simulink model "ride_model"  (R2019a)
settings: Solver=VariableStepAuto  StartTime=0.0  StopTime=120  RelTol=1e-3
libraries: fl_lib x20, nesl_utility x10, eeGeneralControl x1, sdl_lib x1
settings Model: Creator=Owen Heaney  LastModifiedBy=Owen Heaney

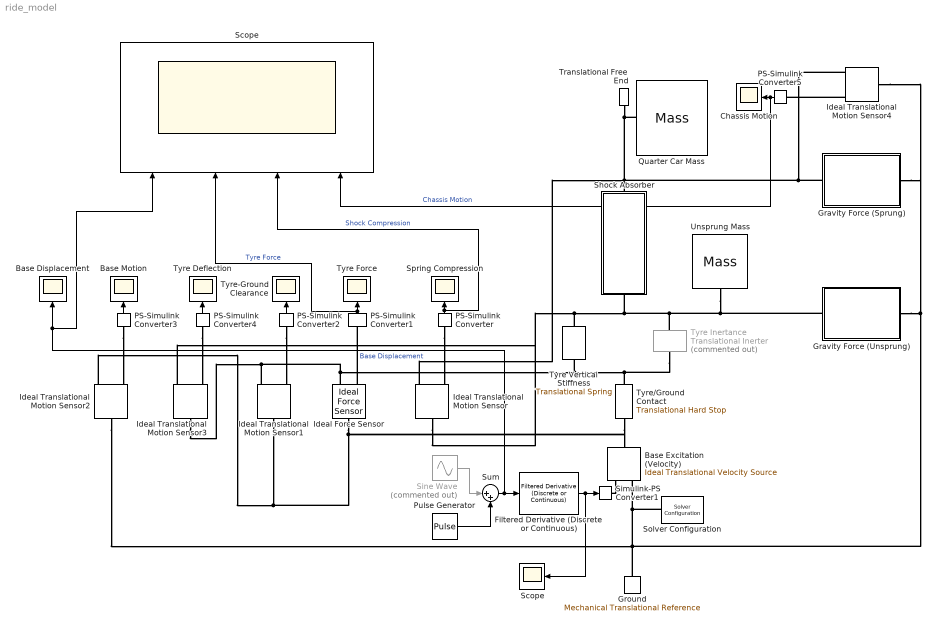
== system ride_model ==
  " Scope" : Scope  NumInputPorts=4
  Base Displacement : Scope
  Base Motion : Scope
  Base Excitation (Velocity) : fl_lib/Mechanical/Mechanical Sources/Ideal Translational Velocity Source
  Chassis Motion : Scope
  Filtered Derivative (Discrete or Continuous) : eeGeneralControl/Filtered Derivative (Discrete or Continuous)  K=1  T=0.0001  B=inf  A=-inf  minRatio=10  Ts=0
      settings: SourceProductName=Simscape Electrical  SourceProductBaseCode=PS
  Gravity Force (Sprung) : Subsystem
  Gravity Force (Unsprung) : Subsystem
  Ground : fl_lib/Mechanical/Translational Elements/Mechanical Translational Reference
  Ideal Force Sensor : fl_lib/Mechanical/Mechanical Sensors/Ideal Force Sensor
  Ideal Translational Motion Sensor{,1..4} (5 alike) : fl_lib/Mechanical/Mechanical Sensors/Ideal Translational Motion Sensor  offset=0 m
  PS-Simulink Converter : nesl_utility/PS-Simulink Converter  PhysicalDomain=network_engine_domain  SubClassName=ps_output  LeftPortType=input  RightPortType=output  PseudoPeriodic=off  Frequencies=[]  Unit=mm  AffineConversion=off
  PS-Simulink Converter{1..4} (4 alike) : nesl_utility/PS-Simulink Converter  PhysicalDomain=network_engine_domain  SubClassName=ps_output  LeftPortType=input  RightPortType=output  PseudoPeriodic=off  Frequencies=[]  Unit=1  AffineConversion=off
  PS-Simulink Converter5 : nesl_utility/PS-Simulink Converter  PhysicalDomain=network_engine_domain  SubClassName=ps_output  LeftPortType=input  RightPortType=output  PseudoPeriodic=off  Frequencies=[]  Unit=mm  AffineConversion=off
  Pulse Generator : DiscretePulseGenerator  PulseType=Time based  Amplitude=0.002  Period=60  PulseWidth=25  PhaseDelay=20
  Quarter Car Mass : fl_lib/Mechanical/Translational Elements/Mass  mass=75 kg  v_specify=off  v_priority=High  v=0 m/s  v_nominal_specify=off  v_nominal_unit=m/s  v_nominal_value=1  f_specify=on  f_priority=None  f=0.01 N  f_nominal_specify=off  f_nominal_unit=N  f_nominal_value=1
  Scope : Scope
  Shock Absorber : Subsystem
  Simulink-PS Converter1 : nesl_utility/Simulink-PS Converter  PhysicalDomain=network_engine_domain  SubClassName=ps_input  LeftPortType=input  RightPortType=output  PseudoPeriodic=off  Frequencies=[]  NoiseDistribution=none  NoiseParameters=[]  Unit=m/s  AffineConversion=off  FilteringAndDerivatives=filter  SimscapeFilterOrder=1  InputFilterTimeConstant=0.001  UdotUserProvided=0
  Sine Wave : Sin  Commented=on  Amplitude=0.001  Frequency=5  SampleTime=0
  Solver Configuration : nesl_utility/Solver Configuration  PhysicalDomain=network_engine_domain  SubClassName=solver  LeftPortType=input  RightPortType=generic  Tones=[]  Harmonics=[]  SimulateNoise=off  Profile=off  UseLocalSampling=off  EnableSwitchedLinearOptims=on  FrequencyDomain=off  UseCCode=off  RelTol=0.001  AbsTol=1e-06  MinStep=1e-09  ToWorkspace=off  RevertToSquareIcSolve=off  NumHomotopyIterations=100  PhasorMode=off  PhasorModeNumHarmonics=1  DoDC=on  ResidualTolerance=1e-15  UseLocalSolver=off  LocalSolverChoice=NE_BACKWARD_EULER_ADVANCER  LocalSolverSampleTime=0.001  DoFixedCost=off  MaxNonlinIter=3  MaxModeIter=2  LinearAlgebra=auto  EquationFormulation=NE_TIME_EF  DelaysMemoryBudget=1024  AutomaticFiltering=on  FilteringTimeConstant=0.001  PartitionStorageMethod=AS_NEEDED  PartitionMemoryBudget=1024  PartitionMethod=ROBUST
  Spring Compression : Scope
  Sum : Sum  Inputs=|++
  Translational Free End : fl_lib/Mechanical/Translational Elements/Translational Free End  v_specify=off  v_priority=None  v=0 m/s  v_nominal_specify=off  v_nominal_unit=m/s  v_nominal_value=1
      settings: SourceProductName=Simscape  SourceProductBaseCode=SS
  Tyre Deflection : Scope
  Tyre Force : Scope
  Tyre Inertance : fl_lib/Mechanical/Translational Elements/Translational Inerter  Commented=on  B=0.001 kg  v_specify=off  v_priority=High  v=0 m/s  v_nominal_specify=off  v_nominal_unit=m/s  v_nominal_value=1  f_specify=off  f_priority=None  f=0 N  f_nominal_specify=off  f_nominal_unit=N  f_nominal_value=1
      settings: SourceProductName=Simscape  SourceProductBaseCode=SS
  Tyre Vertical Stiffness : fl_lib/Mechanical/Translational Elements/Translational Spring  spr_rate=80000 N/m  v_specify=on  v_priority=None  v=0 m/s  v_nominal_specify=off  v_nominal_unit=m/s  v_nominal_value=1  f_specify=off  f_priority=None  f=0 N  f_nominal_specify=off  f_nominal_unit=N  f_nominal_value=1  x_specify=off  x_priority=High  x=0 m  x_nominal_specify=off  x_nominal_unit=m  x_nominal_value=1
  Tyre-Ground Clearance : Scope
  Tyre/Ground Contact : fl_lib/Mechanical/Translational Elements/Translational Hard Stop  upper_bnd=100 m  lower_bnd=0 mm  stiff_up=inf N/m  stiff_low=inf N/m  D_up=inf N/(m/s)  D_low=0 N/(m/s)  model=simscape.enum.hardstop.fullundamped  transition=00.1 mm  v_specify=off  v_priority=None  v=0 m/s  v_nominal_specify=off  v_nominal_unit=m/s  v_nominal_value=1  f_specify=off  f_priority=None  f=0 N  f_nominal_specify=off  f_nominal_unit=N  f_nominal_value=1  x_specify=off  x_priority=High  x=0 m  x_nominal_specify=off  x_nominal_unit=m  x_nominal_value=1
  Unsprung Mass : fl_lib/Mechanical/Translational Elements/Mass  mass=5 kg  v_specify=off  v_priority=High  v=0 m/s  v_nominal_specify=off  v_nominal_unit=m/s  v_nominal_value=1  f_specify=on  f_priority=None  f=-0.01 N  f_nominal_specify=off  f_nominal_unit=N  f_nominal_value=1
  wires:
  PS-Simulink Converter/1 -> " Scope"/3, Spring Compression/1  "Shock Compression"
  PS-Simulink Converter1/1 -> " Scope"/2, Tyre Force/1  "Tyre Force"
  PS-Simulink Converter2/1 -> Tyre-Ground Clearance/1
  PS-Simulink Converter3/1 -> Base Motion/1
  PS-Simulink Converter4/1 -> Tyre Deflection/1
  Filtered Derivative (Discrete or Continuous)/1 -> Scope/1, Simulink-PS Converter1/1
  Sum/1 -> " Scope"/1, Base Displacement/1, Filtered Derivative (Discrete or Continuous)/1  "Base Displacement"
  Pulse Generator/1 -> Sum/2
  Sine Wave/1 -> Sum/1
  PS-Simulink Converter5/1 -> " Scope"/4, Chassis Motion/1  "Chassis Motion"
  connections:
  Gravity Force (Sprung)/LConn1 -- Ideal Translational Motion Sensor4/RConn1 -- Shock Absorber/LConn1 -- Ideal Translational Motion Sensor/RConn1 -- Translational Free End/LConn1 -- Quarter Car Mass/LConn1
  Ideal Translational Motion Sensor2/LConn1 -- Ground/LConn1 -- Ideal Translational Motion Sensor4/LConn1 -- Gravity Force (Sprung)/RConn1 -- Gravity Force (Unsprung)/RConn1 -- Solver Configuration/RConn1 -- Base Excitation (Velocity)/RConn2
  PS-Simulink Converter/LConn1 -- Ideal Translational Motion Sensor/RConn3
  PS-Simulink Converter2/LConn1 -- Ideal Translational Motion Sensor1/RConn3
  PS-Simulink Converter3/LConn1 -- Ideal Translational Motion Sensor2/RConn3
  PS-Simulink Converter4/LConn1 -- Ideal Translational Motion Sensor3/RConn3
  Ideal Force Sensor/RConn1 -- Ideal Translational Motion Sensor3/LConn1 -- Ideal Translational Motion Sensor1/RConn1 -- Tyre Inertance/LConn1 -- Tyre/Ground Contact/LConn1 -- Tyre Vertical Stiffness/LConn1
  Base Excitation (Velocity)/RConn1 -- Simulink-PS Converter1/RConn1
  Ideal Force Sensor/LConn1 -- Tyre/Ground Contact/RConn1 -- Base Excitation (Velocity)/LConn1 -- Ideal Translational Motion Sensor2/RConn1 -- Ideal Translational Motion Sensor1/LConn1
  Gravity Force (Unsprung)/LConn1 -- Unsprung Mass/LConn1 -- Tyre Inertance/RConn1 -- Ideal Translational Motion Sensor/LConn1 -- Ideal Translational Motion Sensor3/RConn1 -- Tyre Vertical Stiffness/RConn1 -- Shock Absorber/RConn1
  Ideal Translational Motion Sensor4/RConn3 -- PS-Simulink Converter5/LConn1
  Ideal Force Sensor/RConn2 -- PS-Simulink Converter1/LConn1

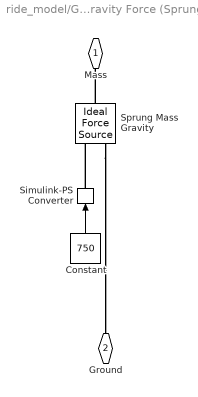
== system ride_model/Gravity Force (Sprung) ==
  Constant : Constant  Value=750
  Simulink-PS Converter : nesl_utility/Simulink-PS Converter  PhysicalDomain=network_engine_domain  SubClassName=ps_input  LeftPortType=input  RightPortType=output  PseudoPeriodic=off  Frequencies=[]  NoiseDistribution=none  NoiseParameters=[]  Unit=1  AffineConversion=off  FilteringAndDerivatives=provide  SimscapeFilterOrder=1  InputFilterTimeConstant=0.001  UdotUserProvided=0
  Sprung Mass Gravity : fl_lib/Mechanical/Mechanical Sources/Ideal Force Source
  Mass : PMIOPort  Side=Left
  Ground : PMIOPort  Port=2  Side=Right
  wires:
  Constant/1 -> Simulink-PS Converter/1
  connections:
  Simulink-PS Converter/RConn1 -- Sprung Mass Gravity/RConn1
  Sprung Mass Gravity/RConn2 -- Ground/RConn1
  Sprung Mass Gravity/LConn1 -- Mass/RConn1

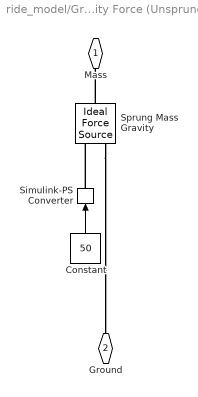
== system ride_model/Gravity Force (Unsprung) ==
  Constant : Constant  Value=50
  Simulink-PS Converter : nesl_utility/Simulink-PS Converter  PhysicalDomain=network_engine_domain  SubClassName=ps_input  LeftPortType=input  RightPortType=output  PseudoPeriodic=off  Frequencies=[]  NoiseDistribution=none  NoiseParameters=[]  Unit=1  AffineConversion=off  FilteringAndDerivatives=provide  SimscapeFilterOrder=1  InputFilterTimeConstant=0.001  UdotUserProvided=0
  Sprung Mass Gravity : fl_lib/Mechanical/Mechanical Sources/Ideal Force Source
  Mass : PMIOPort  Side=Left
  Ground : PMIOPort  Port=2  Side=Right
  wires:
  Constant/1 -> Simulink-PS Converter/1
  connections:
  Sprung Mass Gravity/LConn1 -- Mass/RConn1
  Sprung Mass Gravity/RConn2 -- Ground/RConn1
  Simulink-PS Converter/RConn1 -- Sprung Mass Gravity/RConn1

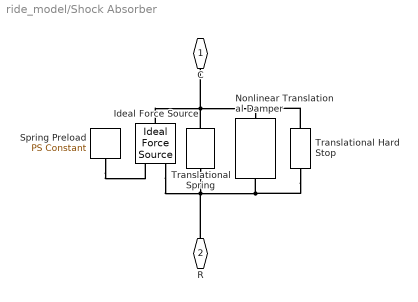
== system ride_model/Shock Absorber ==
  Ideal Force Source : fl_lib/Mechanical/Mechanical Sources/Ideal Force Source
  Nonlinear Translational Damper : sdl_lib/Couplings & Drives/Springs & Dampers/Nonlinear Translational Damper  parameterization=1  symmetry=2  coefficient_vector=[10, 0, 1, 0, .1] N/(m/s)  extension_coefficient_vector=[10, 0, 1, 0, .1] N/(m/s)  contraction_coefficient_vector=[100, -1, 10, 0, 0] N/(m/s)  velocity_vector=[-1, -.5, -.3, -.1, .1, .3, .5, 1] m/s  force_vector=[-100, -40, -20, -5, 5, 20, 40, 100] N  interp_method=simscape.enum.interpolation.linear  extrap_method=simscape.enum.extrapolation.linear
      settings: SourceProductName=Simscape Driveline  SourceProductBaseCode=LD
  Spring Preload : fl_lib/Physical Signals/Sources/PS Constant  constant=100 N
  Translational Hard Stop : fl_lib/Mechanical/Translational Elements/Translational Hard Stop  upper_bnd=0 mm  lower_bnd=-57 mm  stiff_up=1e10 N/m  stiff_low=1e10 N/m  D_up=150 N/(m/s)  D_low=150 N/(m/s)  model=simscape.enum.hardstop.smooth  transition=0.1 mm  v_specify=off  v_priority=None  v=0 m/s  v_nominal_specify=off  v_nominal_unit=m/s  v_nominal_value=1  f_specify=off  f_priority=None  f=0 N  f_nominal_specify=off  f_nominal_unit=N  f_nominal_value=1  x_specify=off  x_priority=High  x=0 m  x_nominal_specify=off  x_nominal_unit=m  x_nominal_value=1
  Translational Spring : fl_lib/Mechanical/Translational Elements/Translational Spring  spr_rate=61294/(1.4^2) N/m  v_specify=on  v_priority=High  v=0 m/s  v_nominal_specify=off  v_nominal_unit=m/s  v_nominal_value=1  f_specify=off  f_priority=None  f=0 N  f_nominal_specify=off  f_nominal_unit=N  f_nominal_value=1  x_specify=off  x_priority=High  x=-25 mm  x_nominal_specify=off  x_nominal_unit=m  x_nominal_value=1
  C : PMIOPort  Side=Left
  R : PMIOPort  Port=2  Side=Right
  connections:
  Ideal Force Source/LConn1 -- C/RConn1 -- Translational Spring/RConn1 -- Translational Hard Stop/RConn1 -- Nonlinear Translational Damper/RConn1
  Spring Preload/RConn1 -- Ideal Force Source/RConn1
  R/RConn1 -- Ideal Force Source/RConn2 -- Translational Hard Stop/LConn1 -- Nonlinear Translational Damper/LConn1 -- Translational Spring/LConn1
